simulink subsystem "Medidor_velocidad"  (R2023b)
settings: Solver=VariableStepAuto  StartTime=0.0  StopTime=10.0  RelTol=1e-3
libraries: arduinosensorlib x2, simulink x1
settings Model: Creator=Felix  LastModifiedBy=Daniel

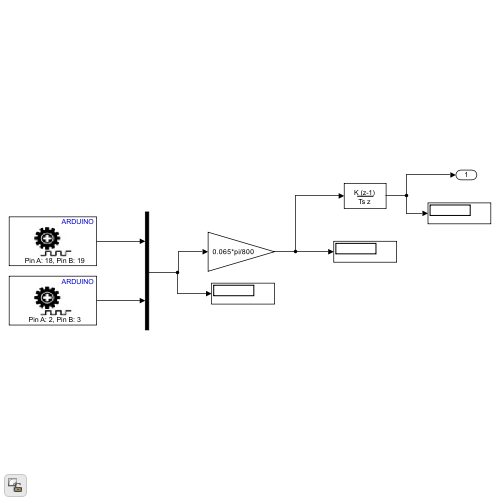
[thumbnail: Simulink's stored preview of the top-level diagram]
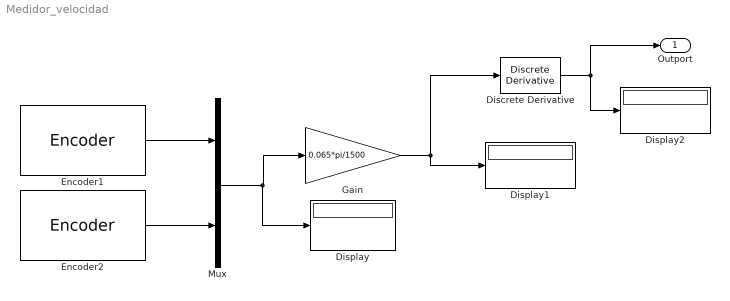
== system Medidor_velocidad ==
  Discrete Derivative : simulink/Discrete/Discrete Derivative  gainval=1.0  ICPrevScaledInput=0.0  OutMin=[]  OutMax=[]  OutDataType=fixdt(1, 16)  OutScaling=2^-10  DoSatur=off
  Display : Display
  Display1 : Display
  Display2 : Display
  Encoder1 : arduinosensorlib/Encoder  InputA=19  InputB=18  Mode=No reset  SampleTime=-1
  Encoder2 : arduinosensorlib/Encoder  InputA=3  InputB=2  Mode=No reset  SampleTime=-1
  Gain : Gain  Gain=0.065*pi/1500  OutDataTypeStr=double
  Mux : Mux  Inputs=2
  Outport : Outport
  wires:
  Gain/1 -> Display1/1, Discrete Derivative/1
  Mux/1 -> Gain/1, Display/1
  Discrete Derivative/1 -> Display2/1, Outport/1
  Encoder1/1 -> Mux/1
  Encoder2/1 -> Mux/2
